simulink model "driver"  (R2023a)
settings: Solver=ode5  StartTime=0.0  StopTime=10.0  RelTol=1e-3
undefined symbols (not defined in the file): canChannel
libraries: canmsglib x4, canlib x3
settings Model: Creator=nineday  LastModifiedBy=nineday
settings HardwareCC: ProdBitPerLong=64  ProdHWDeviceType=Intel->x86-64 (Linux 64)
settings ModelReferenceCC: EnableRefExpFcnMdlSchedulingChecks=on
settings RTWCC: Description=Simulink Desktop Real-Time  SystemTargetFile=sldrt.tlc  TemplateMakefile=sldrt.tmf  RTWCompilerOptimization=on
settings CodeAppCC: MaxIdLength=95
settings SimulinkDesktopRealTimeCC: TargetLibSuffix=_sldrt.a  TargetPreCompLibLocation=D:\A_Work\matlab2023\toolbox\sldrt\lib\win64

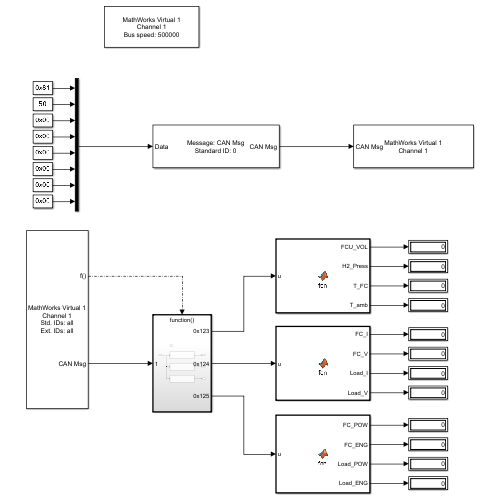
[thumbnail: Simulink's stored preview of the top-level diagram]
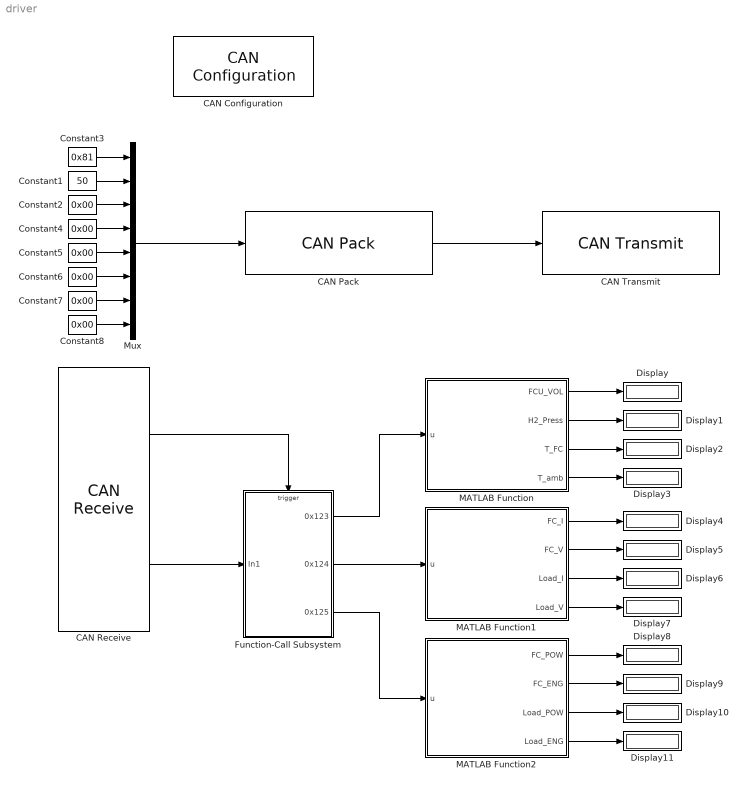
== system driver ==
  CAN Configuration : canlib/CAN Configuration  BlockHandle=2.0001  Device=MathWorks Virtual 1 (Channel 1)  DeviceMenu=MathWorks Virtual 1 (Channel 1)  ObjConstructor=canChannel('MathWorks', 'Virtual 1', 1)  BusSpeed=500000  EnableBitParameters=off  AckMode=Normal
  CAN Pack : canmsglib/CAN Pack  MsgList=(none)  MsgName=CAN Msg  MsgIDType=Standard (11-bit identifier)  MsgIdentifier=0  MsgLength=8  Remote=off  ApplyMinMax=off  BusOutput=off  SignalInfo={}
      settings: DataFormat=raw data
  CAN Receive : canlib/CAN Receive  BlockHandle=6.0001  Device=MathWorks Virtual 1 (Channel 1)  DeviceMenu=MathWorks Virtual 1 (Channel 1)  ObjConstructor=canChannel('MathWorks', 'Virtual 1', 1)  EnableStandardIDsFilter=off  StdIDsCombo=Allow all  StandardIDs=0  EnableExtendedIDsFilter=off  ExtIDsCombo=Allow all  ExtendedIDs=0  SampleTime=0.01  MsgsPerTimestep=all  InternalFilterUpdateStatus=on  BusOutput=off
  CAN Transmit : canlib/CAN Transmit  BlockHandle=9.0001  Device=MathWorks Virtual 1 (Channel 1)  DeviceMenu=MathWorks Virtual 1 (Channel 1)  ObjConstructor=canChannel('MathWorks', 'Virtual 1', 1)  EnableEventTransmit=off  EnablePeriodicTransmit=off  MessagePeriod=1.000
  Constant1 : Constant  Value=50  OutDataTypeStr=uint8
  Constant{2,4..8} (6 alike) : Constant  Value=0x00  OutDataTypeStr=uint8
  Constant3 : Constant  Value=0x81  OutDataTypeStr=uint8
  Display{,1..11} (12 alike) : Display
  Function-Call Subsystem : Subsystem  TreatAsAtomicUnit=on
  MATLAB Function : MATLAB Function  TreatAsAtomicUnit=on
  MATLAB Function1 : MATLAB Function  TreatAsAtomicUnit=on
  MATLAB Function2 : MATLAB Function  TreatAsAtomicUnit=on
  Mux : Mux  Inputs=8
  wires:
  Mux/1 -> CAN Pack/1
  Constant1/1 -> Mux/2
  Constant2/1 -> Mux/3
  Constant4/1 -> Mux/4
  Constant5/1 -> Mux/5
  Constant6/1 -> Mux/6
  Constant7/1 -> Mux/7
  Constant8/1 -> Mux/8
  CAN Pack/1 -> CAN Transmit/1
  CAN Receive/1 -> Function-Call Subsystem/Trigger
  CAN Receive/2 -> Function-Call Subsystem/1(In1)
  Constant3/1 -> Mux/1
  Function-Call Subsystem/1(0x123) -> MATLAB Function/1(u)
  Function-Call Subsystem/2(0x124) -> MATLAB Function1/1(u)
  Function-Call Subsystem/3(0x125) -> MATLAB Function2/1(u)
  MATLAB Function/1(FCU_VOL) -> Display/1
  MATLAB Function/2(H2_Press) -> Display1/1
  MATLAB Function/3(T_FC) -> Display2/1
  MATLAB Function/4(T_amb) -> Display3/1
  MATLAB Function1/1(FC_I) -> Display4/1
  MATLAB Function1/2(FC_V) -> Display5/1
  MATLAB Function1/3(Load_I) -> Display6/1
  MATLAB Function1/4(Load_V) -> Display7/1
  MATLAB Function2/1(FC_POW) -> Display8/1
  MATLAB Function2/2(FC_ENG) -> Display9/1
  MATLAB Function2/3(Load_POW) -> Display10/1
  MATLAB Function2/4(Load_ENG) -> Display11/1

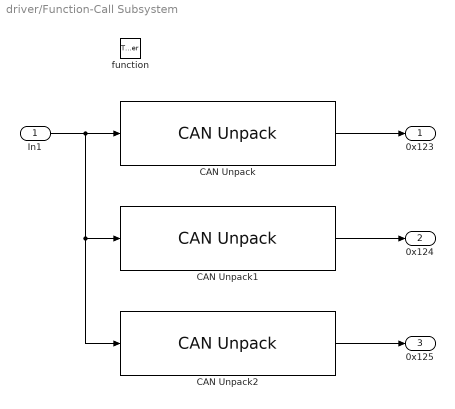
== system driver/Function-Call Subsystem ==
  In1 : Inport
  function : TriggerPort  TriggerType=function-call  VariantControl=(inherit)
  CAN Unpack : canmsglib/CAN Unpack  MsgList=(none)  MsgName=CAN Msg  MsgIDType=Standard (11-bit identifier)  MsgIdentifier=0x123  MsgLength=8  SignalInfo={}  IDPort=off  TimestampPort=off  ErrorPort=off  RemotePort=off  LengthPort=off  StatusPort=off  ApplyMinMax=off
      settings: DataFormat=raw data
  CAN Unpack1 : canmsglib/CAN Unpack  MsgList=(none)  MsgName=CAN Msg  MsgIDType=Standard (11-bit identifier)  MsgIdentifier=0x124  MsgLength=8  SignalInfo={}  IDPort=off  TimestampPort=off  ErrorPort=off  RemotePort=off  LengthPort=off  StatusPort=off  ApplyMinMax=off
      settings: DataFormat=raw data
  CAN Unpack2 : canmsglib/CAN Unpack  MsgList=(none)  MsgName=CAN Msg  MsgIDType=Standard (11-bit identifier)  MsgIdentifier=0x125  MsgLength=8  SignalInfo={}  IDPort=off  TimestampPort=off  ErrorPort=off  RemotePort=off  LengthPort=off  StatusPort=off  ApplyMinMax=off
      settings: DataFormat=raw data
  0x123 : Outport
  0x124 : Outport  Port=2
  0x125 : Outport  Port=3
  wires:
  In1/1 -> CAN Unpack2/1, CAN Unpack1/1, CAN Unpack/1
  CAN Unpack/1 -> 0x123/1
  CAN Unpack1/1 -> 0x124/1
  CAN Unpack2/1 -> 0x125/1

== matlab function driver/MATLAB Function1 ==
  data: u input; FC_I output; FC_V output; Load_I output; Load_V output
function [FC_I, FC_V, Load_I, Load_V] = fcn(u)
FC_I = hex2dec([dec2hex(u(2)), dec2hex(u(1))])/100;
FC_V = hex2dec([dec2hex(u(4)), dec2hex(u(3))])/100;
Load_I = hex2dec([dec2hex(u(6)), dec2hex(u(5))])/100;
Load_V = hex2dec([dec2hex(u(8)), dec2hex(u(7))])/100;

== matlab function driver/MATLAB Function ==
  data: u input; FCU_VOL output; H2_Press output; T_FC output; T_amb output
function [FCU_VOL, H2_Press, T_FC, T_amb] = fcn(u)
FCU_VOL = hex2dec([dec2hex(u(2)), dec2hex(u(1))])/100;
H2_Press = hex2dec([dec2hex(u(4)), dec2hex(u(3))])/100;
T_FC = hex2dec([dec2hex(u(6)), dec2hex(u(5))])/100;
T_amb = hex2dec([dec2hex(u(8)), dec2hex(u(7))])/100;

== matlab function driver/MATLAB Function2 ==
  data: u input; FC_POW output; FC_ENG output; Load_POW output; Load_ENG output
function [FC_POW, FC_ENG, Load_POW, Load_ENG] = fcn(u)
FC_POW = hex2dec([dec2hex(u(2)), dec2hex(u(1))])/100;
FC_ENG = hex2dec([dec2hex(u(4)), dec2hex(u(3))])/100;
Load_POW = hex2dec([dec2hex(u(6)), dec2hex(u(5))])/100;
Load_ENG = hex2dec([dec2hex(u(8)), dec2hex(u(7))])/100;
